simulink model "ControlStudy_model"  (R2022b)
settings: Solver=VariableStepAuto  StartTime=0.0  StopTime=100  RelTol=1e-3
values from neighbouring files (symbols this model uses):
  D_gain_model = 0    [param.m]
  FB_off = false    [param.m]
  I_gain_model = 0    [param.m]
  Limits = 0.2    [param.m]
  Off_dist = 0.1    [param.m]
  P_gain_model = 0    [param.m]
  Sens_delay = 20    [param.m]
  Sens_off = 0    [param.m]
  Sensor_noise = 0.1    [param.m]
  SimEndTime = 10    [param.m]
  System_noise = 0.2    [param.m]
  TimeStep = 0.01    [param.m]
undefined symbols (not defined in the file or in its folder): DiscIntNeverNeededParam
libraries: simulink x5
settings Model: SimulationMode=rapid-accelerator  Creator=pzdz1j  LastModifiedBy=tshintai
settings SolverCC: AlgebraicLoopSolver=TrustRegion
settings OptimizationCC: AccelVerboseBuild=on
settings DebuggingCC: UnconnectedInputMsg=warning  UnconnectedOutputMsg=warning  UnconnectedLineMsg=warning  SFMachineParentedDataDiag=warning
settings ModelReferenceCC: EnableRefExpFcnMdlSchedulingChecks=on
settings RTWCC: DLArmComputeVersion=19.05

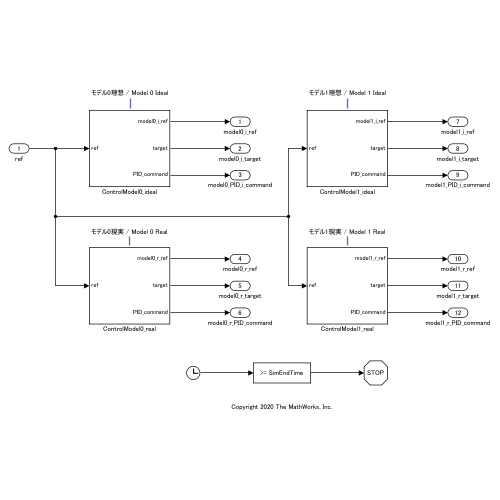
[thumbnail: Simulink's stored preview of the top-level diagram]
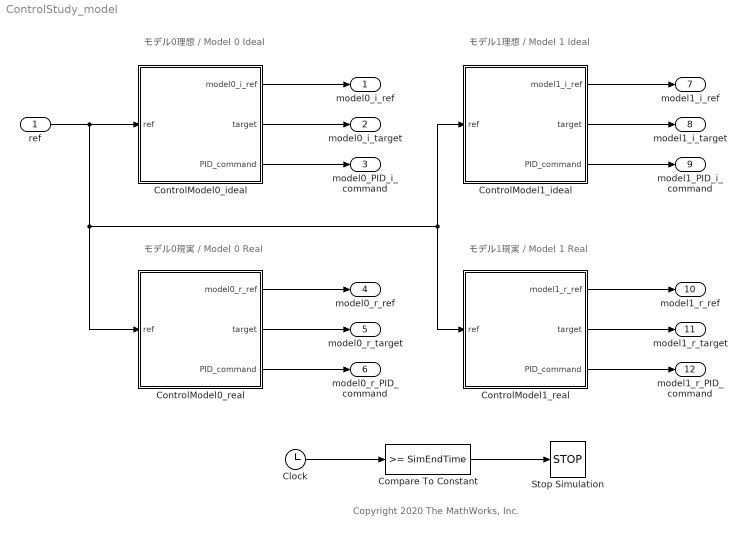
== system ControlStudy_model ==
  note: Copyright 2020 The MathWorks, Inc.
  note: モデル0理想 / Model 0 Ideal
  note: モデル0現実 / Model 0 Real
  note: モデル1理想 / Model 1 Ideal
  note: モデル1現実 / Model 1 Real
  ref : Inport
  Clock : Clock
  Compare To Constant : simulink/Logic and Bit Operations/Compare To Constant  relop=>=  const=SimEndTime  OutDataTypeStr=boolean
  ControlModel0_ideal : Subsystem
  ControlModel0_real : Subsystem
  ControlModel1_ideal : Subsystem
  ControlModel1_real : Subsystem
  Stop Simulation : Stop
  model0_i_ref : Outport
  model0_i_target : Outport  Port=2
  model0_PID_i_command : Outport  Port=3
  model0_r_ref : Outport  Port=4
  model0_r_target : Outport  Port=5
  model0_r_PID_command : Outport  Port=6
  model1_i_ref : Outport  Port=7
  model1_i_target : Outport  Port=8
  model1_PID_i_command : Outport  Port=9
  model1_r_ref : Outport  Port=10
  model1_r_target : Outport  Port=11
  model1_r_PID_command : Outport  Port=12
  wires:
  ControlModel0_ideal/1(model0_i_ref) -> model0_i_ref/1
  ControlModel0_ideal/2(target) -> model0_i_target/1
  ControlModel0_ideal/3(PID_command) -> model0_PID_i_command/1
  ControlModel0_real/1(model0_r_ref) -> model0_r_ref/1
  ControlModel0_real/2(target) -> model0_r_target/1
  ControlModel0_real/3(PID_command) -> model0_r_PID_command/1
  ControlModel1_ideal/1(model1_i_ref) -> model1_i_ref/1
  ControlModel1_ideal/2(target) -> model1_i_target/1
  ControlModel1_ideal/3(PID_command) -> model1_PID_i_command/1
  ControlModel1_real/1(model1_r_ref) -> model1_r_ref/1
  ControlModel1_real/2(target) -> model1_r_target/1
  ControlModel1_real/3(PID_command) -> model1_r_PID_command/1
  Clock/1 -> Compare To Constant/1
  Compare To Constant/1 -> Stop Simulation/1
  ref/1 -> ControlModel1_real/1(ref), ControlModel1_ideal/1(ref), ControlModel0_real/1(ref), ControlModel0_ideal/1(ref)

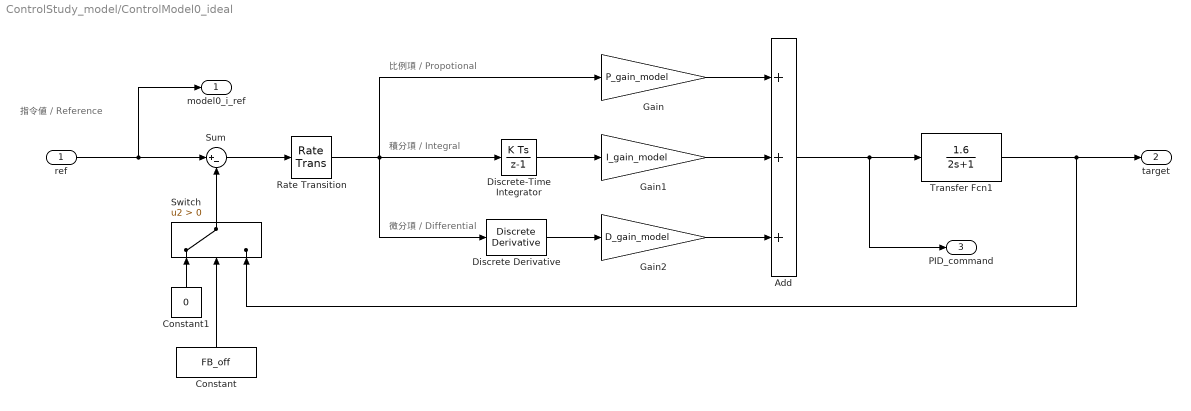
== system ControlStudy_model/ControlModel0_ideal ==
  note: 指令値 / Reference
  note: 積分項 / Integral
  note: 比例項 / Propotional
  note: 微分項 / Differential
  ref : Inport
  Add : Sum  Inputs=+++
  Constant : Constant  Value=FB_off  OutDataTypeStr=boolean
  Constant1 : Constant  Value=0
  Discrete Derivative : simulink/Discrete/Discrete Derivative  gainval=1.0  ICPrevScaledInput=0.0  OutMin=[]  OutMax=[]  OutDataType=fixdt(1, 16)  OutScaling=2^-10  DoSatur=off
  Discrete-Time Integrator : DiscreteIntegrator  SampleTime=-1  ICPrevOutput=DiscIntNeverNeededParam  ICPrevScaledInput=DiscIntNeverNeededParam
  Gain : Gain  Gain=P_gain_model
  Gain1 : Gain  Gain=I_gain_model
  Gain2 : Gain  Gain=D_gain_model
  Rate Transition : RateTransition  OutPortSampleTime=TimeStep
  Sum : Sum  Inputs=|+-
  Switch : Switch  Criteria=u2 > Threshold  SaturateOnIntegerOverflow=off  InputSameDT=off
  Transfer Fcn1 : TransferFcn  Numerator=[1.6]  Denominator=[2 1]
  model0_i_ref : Outport
  target : Outport  Port=2
  PID_command : Outport  Port=3
  wires:
  Transfer Fcn1/1 -> Switch/3, target/1
  Discrete-Time Integrator/1 -> Gain1/1
  Sum/1 -> Rate Transition/1
  Gain1/1 -> Add/2
  Gain2/1 -> Add/3
  Gain/1 -> Add/1
  ref/1 -> model0_i_ref/1, Sum/1
  Discrete Derivative/1 -> Gain2/1
  Add/1 -> PID_command/1, Transfer Fcn1/1
  Rate Transition/1 -> Discrete-Time Integrator/1, Discrete Derivative/1, Gain/1
  Switch/1 -> Sum/2
  Constant/1 -> Switch/2
  Constant1/1 -> Switch/1

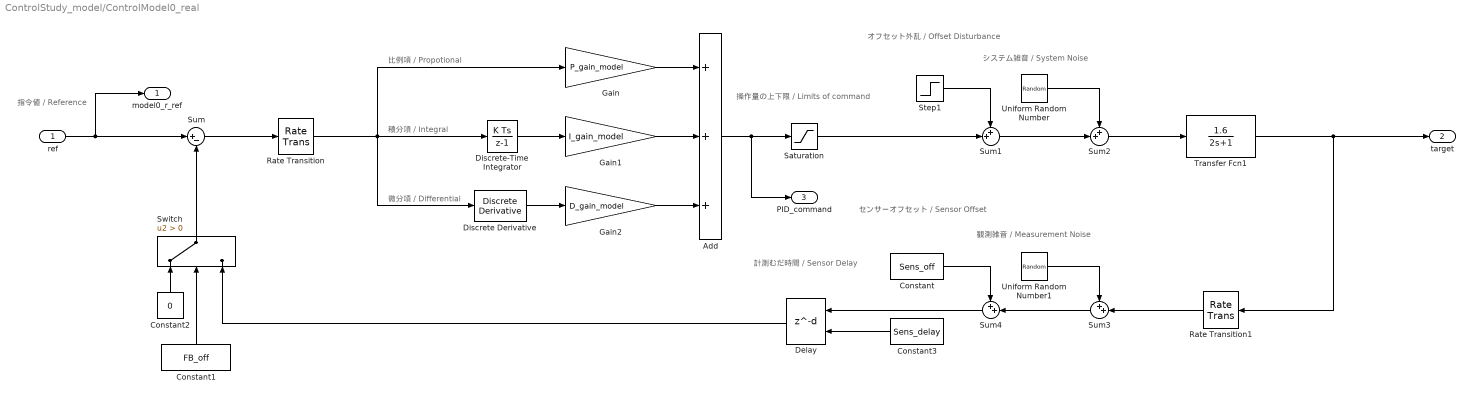
== system ControlStudy_model/ControlModel0_real ==
  note: 計測むだ時間 / Sensor Delay
  note: 操作量の上下限 / Limits of command
  note: システム雑音 / System Noise
  note: オフセット外乱 / Offset Disturbance
  note: 微分項 / Differential
  note: 比例項 / Propotional
  note: 積分項 / Integral
  note: 指令値 / Reference
  note: 観測雑音 / Measurement Noise
  note: センサーオフセット / Sensor Offset
  ref : Inport
  Add : Sum  Inputs=+++
  Constant : Constant  Value=Sens_off
  Constant1 : Constant  Value=FB_off  OutDataTypeStr=boolean
  Constant2 : Constant  Value=0
  Constant3 : Constant  Value=Sens_delay
  Delay : Delay  DelayLengthSource=Input port  DelayLength=Sens_delay
      settings: InputPortMap=u0,p1
  Discrete Derivative : simulink/Discrete/Discrete Derivative  gainval=1.0  ICPrevScaledInput=0.0  OutMin=[]  OutMax=[]  OutDataType=fixdt(1, 16)  OutScaling=2^-10  DoSatur=off
  Discrete-Time Integrator : DiscreteIntegrator  SampleTime=-1  ICPrevOutput=DiscIntNeverNeededParam  ICPrevScaledInput=DiscIntNeverNeededParam
  Gain : Gain  Gain=P_gain_model
  Gain1 : Gain  Gain=I_gain_model
  Gain2 : Gain  Gain=D_gain_model
  Rate Transition : RateTransition  OutPortSampleTime=TimeStep
  Rate Transition1 : RateTransition  OutPortSampleTime=TimeStep
  Saturation : Saturate  UpperLimit=Limits  LowerLimit=-Limits
  Step1 : Step  Time=5  After=Off_dist  SampleTime=TimeStep
  Sum : Sum  Inputs=|+-
  Sum{1..4} (4 alike) : Sum  Inputs=++|
  Switch : Switch  Criteria=u2 > Threshold  SaturateOnIntegerOverflow=off  InputSameDT=off
  Transfer Fcn1 : TransferFcn  Numerator=[1.6]  Denominator=[2 1]
  Uniform Random Number : UniformRandomNumber  Minimum=-System_noise  Maximum=System_noise  SampleTime=TimeStep
  Uniform Random Number1 : UniformRandomNumber  Minimum=-Sensor_noise  Maximum=Sensor_noise  Seed=1  SampleTime=TimeStep
  model0_r_ref : Outport
  target : Outport  Port=2
  PID_command : Outport  Port=3
  wires:
  Discrete Derivative/1 -> Gain2/1
  ref/1 -> model0_r_ref/1, Sum/1
  Sum2/1 -> Transfer Fcn1/1
  Gain/1 -> Add/1
  Gain2/1 -> Add/3
  Gain1/1 -> Add/2
  Sum/1 -> Rate Transition/1
  Discrete-Time Integrator/1 -> Gain1/1
  Transfer Fcn1/1 -> target/1, Rate Transition1/1
  Step1/1 -> Sum1/1
  Sum1/1 -> Sum2/2
  Uniform Random Number/1 -> Sum2/1
  Saturation/1 -> Sum1/2
  Sum4/1 -> Delay/1
  Uniform Random Number1/1 -> Sum3/1
  Sum3/1 -> Sum4/2
  Constant/1 -> Sum4/1
  Add/1 -> PID_command/1, Saturation/1
  Delay/1 -> Switch/3
  Rate Transition/1 -> Discrete-Time Integrator/1, Discrete Derivative/1, Gain/1
  Rate Transition1/1 -> Sum3/2
  Constant2/1 -> Switch/1
  Constant1/1 -> Switch/2
  Switch/1 -> Sum/2
  Constant3/1 -> Delay/2

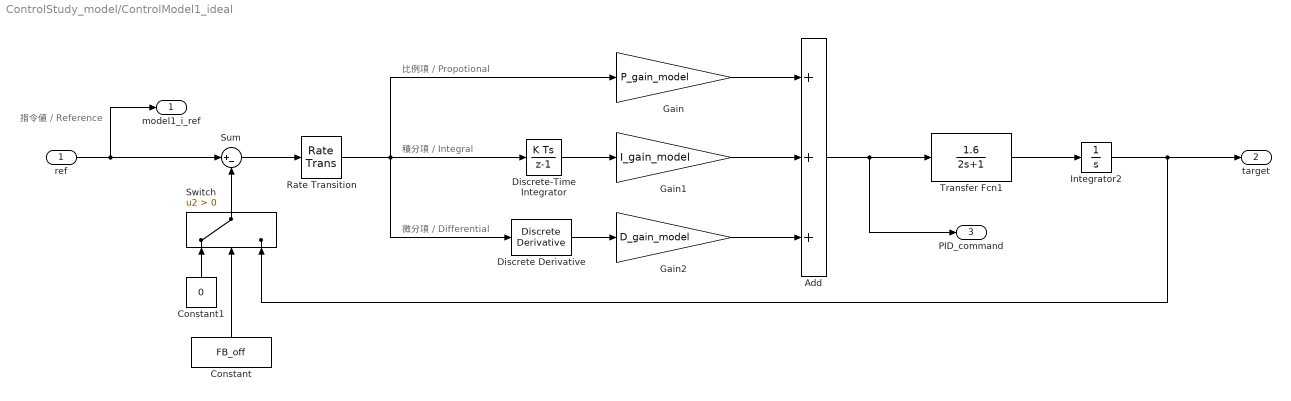
== system ControlStudy_model/ControlModel1_ideal ==
  note: 微分項 / Differential
  note: 比例項 / Propotional
  note: 積分項 / Integral
  note: 指令値 / Reference
  ref : Inport
  Add : Sum  Inputs=+++
  Constant : Constant  Value=FB_off  OutDataTypeStr=boolean
  Constant1 : Constant  Value=0
  Discrete Derivative : simulink/Discrete/Discrete Derivative  gainval=1.0  ICPrevScaledInput=0.0  OutMin=[]  OutMax=[]  OutDataType=fixdt(1, 16)  OutScaling=2^-10  DoSatur=off
  Discrete-Time Integrator : DiscreteIntegrator  SampleTime=-1  ICPrevOutput=DiscIntNeverNeededParam  ICPrevScaledInput=DiscIntNeverNeededParam
  Gain : Gain  Gain=P_gain_model
  Gain1 : Gain  Gain=I_gain_model
  Gain2 : Gain  Gain=D_gain_model
  Integrator2 : Integrator
  Rate Transition : RateTransition  OutPortSampleTime=TimeStep
  Sum : Sum  Inputs=|+-
  Switch : Switch  Criteria=u2 > Threshold  SaturateOnIntegerOverflow=off  InputSameDT=off
  Transfer Fcn1 : TransferFcn  Numerator=[1.6]  Denominator=[2 1]
  model1_i_ref : Outport
  target : Outport  Port=2
  PID_command : Outport  Port=3
  wires:
  Discrete Derivative/1 -> Gain2/1
  ref/1 -> model1_i_ref/1, Sum/1
  Add/1 -> PID_command/1, Transfer Fcn1/1
  Gain/1 -> Add/1
  Gain2/1 -> Add/3
  Gain1/1 -> Add/2
  Sum/1 -> Rate Transition/1
  Discrete-Time Integrator/1 -> Gain1/1
  Integrator2/1 -> Switch/3, target/1
  Transfer Fcn1/1 -> Integrator2/1
  Rate Transition/1 -> Discrete-Time Integrator/1, Discrete Derivative/1, Gain/1
  Constant1/1 -> Switch/1
  Constant/1 -> Switch/2
  Switch/1 -> Sum/2

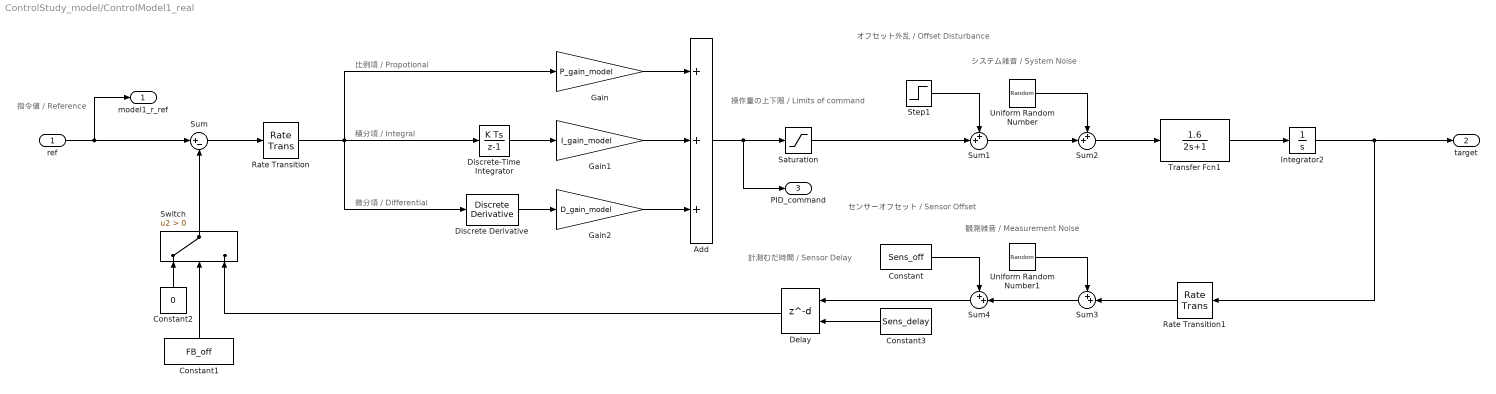
== system ControlStudy_model/ControlModel1_real ==
  note: 指令値 / Reference
  note: 積分項 / Integral
  note: 比例項 / Propotional
  note: 微分項 / Differential
  note: 計測むだ時間 / Sensor Delay
  note: 操作量の上下限 / Limits of command
  note: システム雑音 / System Noise
  note: オフセット外乱 / Offset Disturbance
  note: 観測雑音 / Measurement Noise
  note: センサーオフセット / Sensor Offset
  ref : Inport
  Add : Sum  Inputs=+++
  Constant : Constant  Value=Sens_off
  Constant1 : Constant  Value=FB_off  OutDataTypeStr=boolean
  Constant2 : Constant  Value=0
  Constant3 : Constant  Value=Sens_delay
  Delay : Delay  DelayLengthSource=Input port  DelayLength=Sens_delay
      settings: InputPortMap=u0,p1
  Discrete Derivative : simulink/Discrete/Discrete Derivative  gainval=1.0  ICPrevScaledInput=0.0  OutMin=[]  OutMax=[]  OutDataType=fixdt(1, 16)  OutScaling=2^-10  DoSatur=off
  Discrete-Time Integrator : DiscreteIntegrator  SampleTime=-1  ICPrevOutput=DiscIntNeverNeededParam  ICPrevScaledInput=DiscIntNeverNeededParam
  Gain : Gain  Gain=P_gain_model
  Gain1 : Gain  Gain=I_gain_model
  Gain2 : Gain  Gain=D_gain_model
  Integrator2 : Integrator
  Rate Transition : RateTransition  OutPortSampleTime=TimeStep
  Rate Transition1 : RateTransition  OutPortSampleTime=TimeStep
  Saturation : Saturate  UpperLimit=Limits  LowerLimit=-Limits
  Step1 : Step  Time=20  After=Off_dist  SampleTime=TimeStep
  Sum : Sum  Inputs=|+-
  Sum{1..4} (4 alike) : Sum  Inputs=++|
  Switch : Switch  Criteria=u2 > Threshold  SaturateOnIntegerOverflow=off  InputSameDT=off
  Transfer Fcn1 : TransferFcn  Numerator=[1.6]  Denominator=[2 1]
  Uniform Random Number : UniformRandomNumber  Minimum=-System_noise  Maximum=System_noise  SampleTime=TimeStep
  Uniform Random Number1 : UniformRandomNumber  Minimum=-Sensor_noise  Maximum=Sensor_noise  Seed=1  SampleTime=TimeStep
  model1_r_ref : Outport
  target : Outport  Port=2
  PID_command : Outport  Port=3
  wires:
  Discrete-Time Integrator/1 -> Gain1/1
  Sum/1 -> Rate Transition/1
  Gain1/1 -> Add/2
  Gain2/1 -> Add/3
  Gain/1 -> Add/1
  ref/1 -> model1_r_ref/1, Sum/1
  Discrete Derivative/1 -> Gain2/1
  Step1/1 -> Sum1/1
  Sum1/1 -> Sum2/2
  Uniform Random Number/1 -> Sum2/1
  Saturation/1 -> Sum1/2
  Sum4/1 -> Delay/1
  Uniform Random Number1/1 -> Sum3/1
  Sum3/1 -> Sum4/2
  Constant/1 -> Sum4/1
  Add/1 -> PID_command/1, Saturation/1
  Delay/1 -> Switch/3
  Sum2/1 -> Transfer Fcn1/1
  Integrator2/1 -> target/1, Rate Transition1/1
  Transfer Fcn1/1 -> Integrator2/1
  Rate Transition/1 -> Discrete-Time Integrator/1, Discrete Derivative/1, Gain/1
  Rate Transition1/1 -> Sum3/2
  Constant2/1 -> Switch/1
  Constant1/1 -> Switch/2
  Switch/1 -> Sum/2
  Constant3/1 -> Delay/2
